simulink model "Helicopter"  (Simulink 5.0)
settings: Solver=ode5  StartTime=0.0  StopTime=200  FixedStep=dt  RelTol=1e-3
PreLoadFcn:
  | load HelicopterData
InitFcn:
  | ;fxptdlg('fxptdlg_simInit_cb');
StartFcn:
  | ;fxptdlg('fxptdlg_sim_cb');
StopFcn:
  | ;fxptdlg('fxptdlg_store_cb');
values from neighbouring files (symbols this model uses):
  mr_offset = [1.47 0 0.2]    [HELICOPT.MAT]    (also in MODELPAR.M)
  ned_pos_to_vr = [0  0  -1; 1  0  0; 0  -1  0]    [HELICOPT.MAT]    (also in MODELPAR.M = [0 0 -1; 1 0 0; 0 -1 0])
  ned_rot_to_vr = [0 1 0 0 0 0 -1 0 -1 0 0 0 ... (16 elements, 4x4)]    [HELICOPT.MAT]    (also in MODELPAR.M = [0 0 -1 0; 1 0 0 0; 0 -1 0 0; 0 0 0 1])
  tr_offset = [-4.88 0 -1.36]    [HELICOPT.MAT]    (also in MODELPAR.M)
libraries: dnglibv1 x12, fixpt_lib_4 x4, simulink x3, mblibv1 x3, HelicopterBlockset x2, vrlib x1
PreSaveFcn:
  | ;fxptdlg('fxptdlg_presave_cb');
CloseFcn:
  | ;fxptdlg('fxptdlg_close_cb');
settings Model: MinMaxOverflowLogging=MinMaxAndOverflow  LastModifiedBy=Jim  ExtModeMexFile=ext_xpc  ExtModeArmWhenConnect=off  SaveTime=off  SaveOutput=off  ConsistencyChecking=warning  ArrayBoundsChecking=warning  SingleTaskRateTransMsg=warning  CheckForMatrixSingularity=warning  UnnecessaryDatatypeConvMsg=warning  SignalLabelMismatchMsg=warning  SfunCompatibilityCheckMsg=warning  OptimizeBlockIOStorage=off  RTWSystemTargetFile=xpctarget.tlc  RTWTemplateMakefile=xpc_default_tmf  RTWOptions="-aEnforceIntegerDowncast=0 -aExtMode=1 -aFoldNonRolledExpr=0 -aForceParamTrailComments=0 -aGenerateComments=1 -aGenerateReport=1 -aIncDataTypeInIds=0 -aIncHierarchyInIds=0 -aInlineInvariantSignals=0 -aInlinedPrmAccess=\"Literals\" -aLocalBlockOutputs=0 -aMaxRTWIdLen=31 -aPrefixModelToSubsysFcnNames=1 -aRL32IRQSourceModifier=\"Timer\" -aRL32LogBufSizeModifier=100000 -aRL32LogTETModifier=1 -aRL32ModeModifier=\"Real-Time\" -aRL32ObjectName=\"tg\" -aRTWVerbose=1 -aRollThreshold=5 -aShowEliminatedStatements=0 -axPCIOIRQSlot=-1 -axPCIRQSourceBoard=\"None/Other\" -axpcDblBuff=0 -axpcObjCom=0"

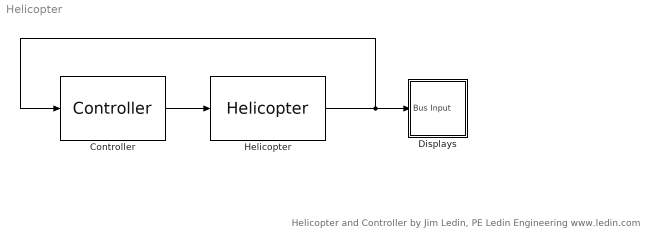
== system Helicopter ==
  note: Helicopter and Controller
      | by Jim Ledin, PE
      | Ledin Engineering
      | www.ledin.com
  Controller : HelicopterBlockset/Controller  TreatAsAtomicUnit=on  SimViewingDevice=off  DataTypeOverride=UseLocalSettings  MinMaxOverflowLogging=UseLocalSettings
      settings: Permissions=ReadWrite  RTWFcnNameOpts=Auto  RTWFileNameOpts=Auto
  Displays : Subsystem
  Helicopter : HelicopterBlockset/Helicopter  SimViewingDevice=off  DataTypeOverride=UseLocalSettings  MinMaxOverflowLogging=UseLocalSettings
      settings: Permissions=ReadWrite  RTWFcnNameOpts=Auto  RTWFileNameOpts=Auto
  wires:
  Helicopter/1 -> Controller/1, Displays/1(Bus Input)
  Controller/1 -> Helicopter/1

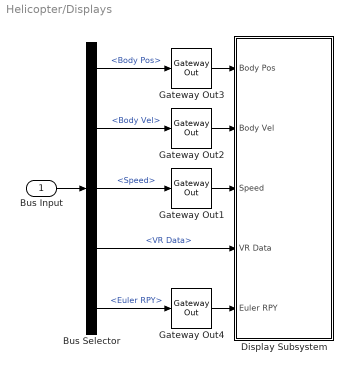
== system Helicopter/Displays ==
  Bus Input : Inport
  Bus Selector : BusSelector  OutputSignals=Body Pos,Body Vel,Speed,VR Data,Euler RPY
  Display Subsystem : Subsystem
  Gateway Out{1..4} (4 alike) : fixpt_lib_4/Data Type/Gateway Out  OutRealWorld=Real World Value  OutBuiltInType=double  RndMeth=Nearest  DoSatur=off
  wires:
  Bus Selector/1 -> Gateway Out3/1  "<Body Pos>"
  Bus Selector/2 -> Gateway Out2/1  "<Body Vel>"
  Bus Selector/3 -> Gateway Out1/1  "<Speed>"
  Bus Selector/4 -> Display Subsystem/4(VR Data)  "<VR Data>"
  Bus Selector/5 -> Gateway Out4/1  "<Euler RPY>"
  Bus Input/1 -> Bus Selector/1
  Gateway Out4/1 -> Display Subsystem/5(Euler RPY)
  Gateway Out1/1 -> Display Subsystem/3(Speed)
  Gateway Out2/1 -> Display Subsystem/2(Body Vel)
  Gateway Out3/1 -> Display Subsystem/1(Body Pos)

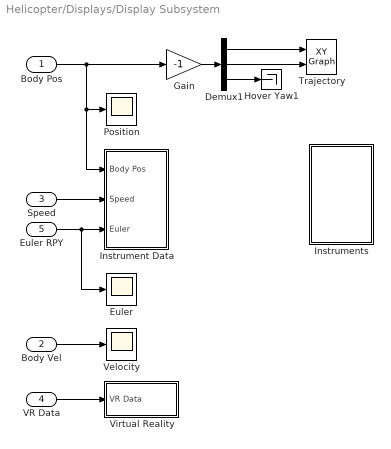
== system Helicopter/Displays/Display Subsystem ==
  Body Pos : Inport
  Body Vel : Inport  Port=2
  Speed : Inport  Port=3
  VR Data : Inport  Port=4
  Euler RPY : Inport  Port=5
  Demux1 : Demux  Outputs=3
  Euler : Scope
      settings: TimeRange=200  YMin=-10  YMax=10
  Gain : Gain  Gain=-1  SaturateOnIntegerOverflow=on
  Hover Yaw1 : Terminator
  Instrument Data : Subsystem
  Instruments : Subsystem
  Position : Scope
      settings: TimeRange=200  YMin=-200  YMax=200
  Trajectory : simulink/Sinks/XY Graph  xmin=-10  xmax=210  ymin=-10  ymax=210  st=-1
  Velocity : Scope
      settings: TimeRange=200  YMin=-10  YMax=10  SaveName=ScopeData2
  Virtual Reality : Subsystem
  wires:
  Demux1/3 -> Hover Yaw1/1
  Demux1/1 -> Trajectory/1
  Demux1/2 -> Trajectory/2
  Gain/1 -> Demux1/1
  Body Vel/1 -> Velocity/1
  Euler RPY/1 -> Euler/1, Instrument Data/3(Euler)
  Speed/1 -> Instrument Data/2(Speed)
  VR Data/1 -> Virtual Reality/1(VR Data)
  Body Pos/1 -> Instrument Data/1(Body Pos), Position/1, Gain/1

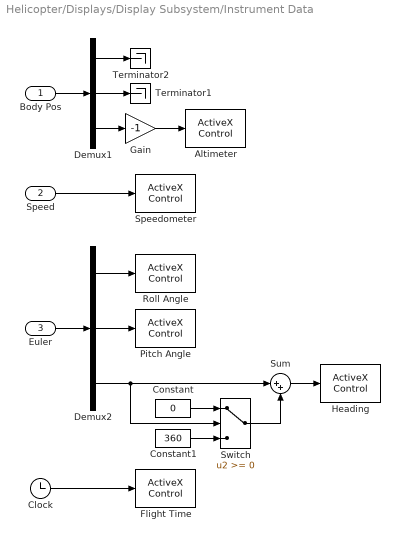
== system Helicopter/Displays/Display Subsystem/Instrument Data ==
  Body Pos : Inport
  Speed : Inport  Port=2
  Euler : Inport  Port=3
  Altimeter : dnglibv1/ActiveX Control  Tag=010  progid=Compass  connect=input  input=Value  init_fcn=Helicopter/Displays/Display Subsystem/Instruments/Altitude (m)  inblock=off  border=on  dialOut=0  updateParam=0
  Clock : Clock
      settings: Decimation=10
  Constant : Constant  Value=0
  Constant1 : Constant  Value=360
  Demux1 : Demux  Outputs=3
  Demux2 : Demux  Outputs=3
  Flight Time : dnglibv1/ActiveX Control  Tag=010  progid=Compass  connect=input  input=Value  init_fcn=Helicopter/Displays/Display Subsystem/Instruments/Flight Time (sec)  inblock=off  border=on  dialOut=0  updateParam=0
  Gain : Gain  Gain=-1  SaturateOnIntegerOverflow=on
  Heading : dnglibv1/ActiveX Control  Tag=010  progid=Compass  connect=input  input=NeedleValue  init_fcn=Helicopter/Displays/Display Subsystem/Instruments/Heading (deg true)  inblock=off  border=on  dialOut=0  updateParam=0
  Pitch Angle : dnglibv1/ActiveX Control  Tag=010  progid=Compass  connect=input  input=NeedleValue  init_fcn=Helicopter/Displays/Display Subsystem/Instruments/Pitch Angle (deg)  inblock=off  border=on  dialOut=0  updateParam=0
  Roll Angle : dnglibv1/ActiveX Control  Tag=010  progid=Compass  connect=input  input=NeedleValue  init_fcn=Helicopter/Displays/Display Subsystem/Instruments/Roll Angle (deg)  inblock=off  border=on  dialOut=0  updateParam=0
  Speedometer : dnglibv1/ActiveX Control  Tag=010  progid=Compass  connect=input  input=Value  init_fcn=Helicopter/Displays/Display Subsystem/Instruments/Speed (m//sec)  inblock=off  border=on  dialOut=0  updateParam=0
  Sum : Sum  Inputs=|++  SaturateOnIntegerOverflow=on
  Switch : Switch  SaturateOnIntegerOverflow=on
  Terminator1 : Terminator
  Terminator2 : Terminator
  wires:
  Euler/1 -> Demux2/1
  Demux2/3 -> Switch/2, Sum/1
  Demux2/1 -> Roll Angle/1
  Demux2/2 -> Pitch Angle/1
  Clock/1 -> Flight Time/1
  Demux1/1 -> Terminator2/1
  Demux1/2 -> Terminator1/1
  Body Pos/1 -> Demux1/1
  Demux1/3 -> Gain/1
  Gain/1 -> Altimeter/1
  Constant/1 -> Switch/1
  Constant1/1 -> Switch/3
  Switch/1 -> Sum/2
  Speed/1 -> Speedometer/1
  Sum/1 -> Heading/1

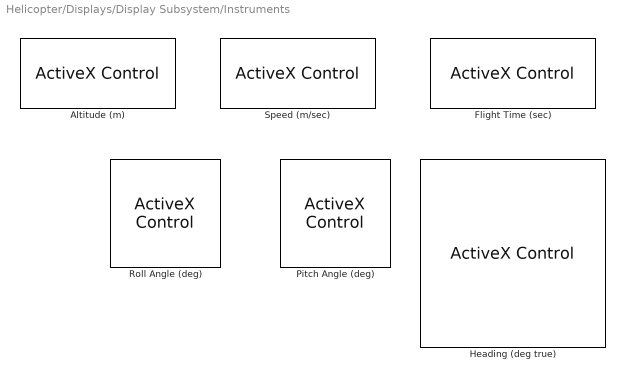
== system Helicopter/Displays/Display Subsystem/Instruments ==
  Altitude (m) : dnglibv1/ActiveX Control  progid=mwnumled.numledctrl.1  connect=neither  input=Value  init=hActx.configuration='Numeric LED\PlusMinus XX.XXX';hActx.Digits=6;hActx.Decimals=3;hActx.FixedDecimal=1;hActx.value=-317.489;hActx.SegmentWidth=3;  inblock=on  border=on  dialOut=0  updateParam=0
  Flight Time (sec) : dnglibv1/ActiveX Control  progid=mwnumled.numledctrl.1  connect=neither  input=Value  init=hActx.Digits=6;hActx.Decimals=2;hActx.FixedDecimal=1;hActx.value=1234.56;  inblock=on  border=on  dialOut=0  updateParam=0
  Heading (deg true) : dnglibv1/ActiveX Control  progid=mwagauge.agaugectrl.1  connect=neither  input=NeedleValue  init=hActx.configuration='Angular Gauge\Compass';  inblock=on  border=on  dialOut=0  updateParam=0
  Pitch Angle (deg) : dnglibv1/ActiveX Control  progid=mwagauge.agaugectrl.1  connect=neither  input=NeedleValue  inblock=on  border=on  dialOut=0  updateParam=0
  Roll Angle (deg) : dnglibv1/ActiveX Control  progid=mwagauge.agaugectrl.1  connect=neither  input=NeedleValue  inblock=on  border=on  dialOut=0  updateParam=0
  Speed (m/sec) : dnglibv1/ActiveX Control  progid=mwnumled.numledctrl.1  connect=neither  input=Value  init=hActx.configuration='Numeric LED\PlusMinus XX.XXX';hActx.Digits=6;hActx.Decimals=3;hActx.FixedDecimal=1;hActx.value=-317.489;hActx.SegmentWidth=3;  inblock=on  border=on  dialOut=0  updateParam=0

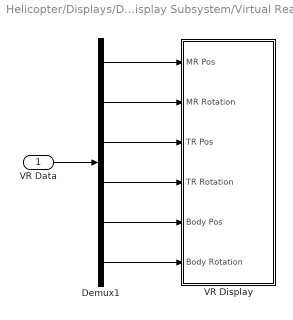
== system Helicopter/Displays/Display Subsystem/Virtual Reality ==
  VR Data : Inport
  Demux1 : Demux  Outputs=[3 9 3 9 3 9]
  VR Display : Subsystem
  wires:
  VR Data/1 -> Demux1/1
  Demux1/1 -> VR Display/1(MR Pos)
  Demux1/2 -> VR Display/2(MR Rotation)
  Demux1/3 -> VR Display/3(TR Pos)
  Demux1/4 -> VR Display/4(TR Rotation)
  Demux1/5 -> VR Display/5(Body Pos)
  Demux1/6 -> VR Display/6(Body Rotation)

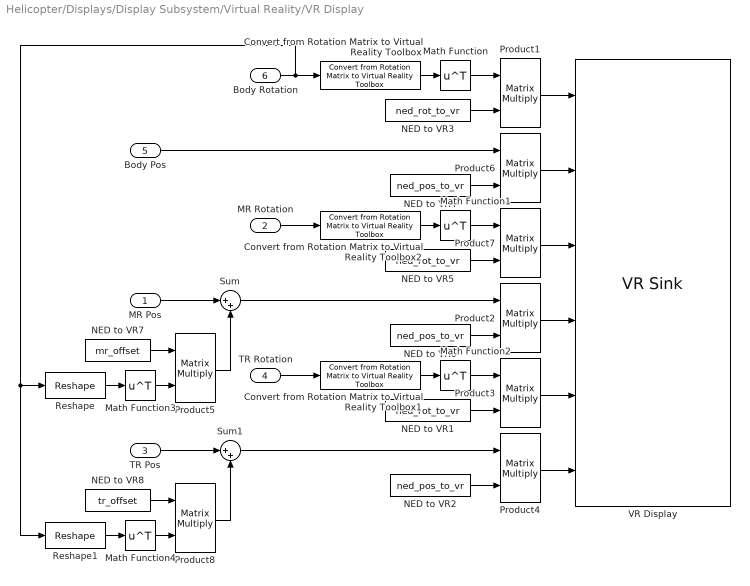
== system Helicopter/Displays/Display Subsystem/Virtual Reality/VR Display ==
  MR Pos : Inport
  MR Rotation : Inport  Port=2
  TR Pos : Inport  Port=3
  TR Rotation : Inport  Port=4
  Body Pos : Inport  Port=5
  Body Rotation : Inport  Port=6
  Convert from Rotation Matrix to Virtual Reality Toolbox : mblibv1/Utilities/Convert from Rotation Matrix to Virtual Reality Toolbox  Tag=Pose2VR
  Convert from Rotation Matrix to Virtual Reality Toolbox1 : mblibv1/Utilities/Convert from Rotation Matrix to Virtual Reality Toolbox  Tag=Pose2VR
  Convert from Rotation Matrix to Virtual Reality Toolbox2 : mblibv1/Utilities/Convert from Rotation Matrix to Virtual Reality Toolbox  Tag=Pose2VR
  Math Function{,1..4} (5 alike) : Math  Operator=transpose
  NED to VR1 : Constant  Value=ned_rot_to_vr
  NED to VR2 : Constant  Value=ned_pos_to_vr
  NED to VR3 : Constant  Value=ned_rot_to_vr
  NED to VR4 : Constant  Value=ned_pos_to_vr
  NED to VR5 : Constant  Value=ned_rot_to_vr
  NED to VR6 : Constant  Value=ned_pos_to_vr
  NED to VR7 : Constant  Value=mr_offset  VectorParams1D=off
  NED to VR8 : Constant  Value=tr_offset  VectorParams1D=off
  Product{1..8} (8 alike) : Product  Multiplication=Matrix(*)  SaturateOnIntegerOverflow=on
  Reshape : simulink/Math Operations/Reshape  OutputDimensionality=Customize  OutputDimensions=[3,3]
  Reshape1 : simulink/Math Operations/Reshape  OutputDimensionality=Customize  OutputDimensions=[3,3]
  Sum : Sum  Inputs=|++  SaturateOnIntegerOverflow=on
  Sum1 : Sum  Inputs=|++  SaturateOnIntegerOverflow=on
  VR Display : vrlib/VR Sink  SampleTime=-1  ViewEnable=on  RemoteChange=off  RemoteView=off  FieldsWritten=Helicopter.rotation.4#Helicopter.translation.3#Main_Rotor.rotation.4#Main_Rotor.translation.3#Tail_Rotor.rotation.4#Tail_Rotor.translation.3  WorldFileName=helicopter_runway.WRL  WorldDescription=Helicopter  AutoView=on  FigureProperties="{'Position', 'Name', 'Viewpoint', 'CameraBound', 'CameraDirection', 'CameraPosition', 'CameraUpVector', 'ZoomFactor', 'Antialiasing', 'Headlight', 'Lighting', 'PanelMode', 'Textures', 'Transparency', 'Wireframe', 'NavZones', 'InfoStrip', 'NavMode', 'NavSpeed', ; [5.0000000000000000e+000  2.5000000000000000e+001  4.0000000000000000e+002  3.2000000000000000e+002], 'Helicopter', 'Observe Helicopter', 'on', [6.2511840616084752e-002 -9.4108294567115919e-002 -9.9359745303440561e-001], [0.0000000000000000e+000  0.0000000000000000e+000  0.0000000000000000e+000], [0.0000000000000000e+000  1.0000000000000000e+000  0.0000000000000000e+000], [1.0000000000000000e+000], 'off', 'on', 'on', 'halfbar', 'on', 'on', 'off', 'off', 'off', 'fly', 'normal', ; }"
  wires:
  Convert from Rotation Matrix to Virtual Reality Toolbox2/1 -> Math Function1/1
  TR Rotation/1 -> Convert from Rotation Matrix to Virtual Reality Toolbox1/1
  MR Rotation/1 -> Convert from Rotation Matrix to Virtual Reality Toolbox2/1
  Body Rotation/1 -> Convert from Rotation Matrix to Virtual Reality Toolbox/1, Reshape/1, Reshape1/1
  Convert from Rotation Matrix to Virtual Reality Toolbox/1 -> Math Function/1
  Math Function/1 -> Product1/1
  Math Function1/1 -> Product7/1
  Body Pos/1 -> Product6/1
  Math Function2/1 -> Product3/1
  Convert from Rotation Matrix to Virtual Reality Toolbox1/1 -> Math Function2/1
  NED to VR3/1 -> Product1/2
  NED to VR4/1 -> Product6/2
  NED to VR5/1 -> Product7/2
  NED to VR6/1 -> Product2/2
  NED to VR1/1 -> Product3/2
  NED to VR2/1 -> Product4/2
  MR Pos/1 -> Sum/1
  Sum/1 -> Product2/1
  NED to VR7/1 -> Product5/1
  Product5/1 -> Sum/2
  Reshape/1 -> Math Function3/1
  Math Function3/1 -> Product5/2
  NED to VR8/1 -> Product8/1
  Product8/1 -> Sum1/2
  Reshape1/1 -> Math Function4/1
  Math Function4/1 -> Product8/2
  Sum1/1 -> Product4/1
  TR Pos/1 -> Sum1/1
  Product1/1 -> VR Display/1
  Product6/1 -> VR Display/2
  Product7/1 -> VR Display/3
  Product2/1 -> VR Display/4
  Product3/1 -> VR Display/5
  Product4/1 -> VR Display/6
